simulink model "servomotor_pi_discreto"  (R2022b)
settings: Solver=FixedStepAuto  StartTime=0.0  StopTime=tempoSimulacao  FixedStep=1e-4  RelTol=1e-3
values from neighbouring files (symbols this model uses):
  controlador = projetarControladorPI(planta, requisitos)    [avaliarIndutor.m]    (also in avaliarTempoSubida.m)
  planta = obterPlantaServo()    [avaliarIndutor.m]    (also in avaliarTempoSubida.m)
undefined symbols (not defined in the file or in its folder): disturbio, referencia
settings Model: Creator=mmaximo  LastModifiedBy=danie
settings SolverCC: AlgebraicLoopSolver=TrustRegion
settings DebuggingCC: UnconnectedInputMsg=warning  UnconnectedOutputMsg=warning  UnconnectedLineMsg=warning  SFMachineParentedDataDiag=warning
settings ModelReferenceCC: EnableRefExpFcnMdlSchedulingChecks=on
settings RTWCC: DLArmComputeVersion=19.05

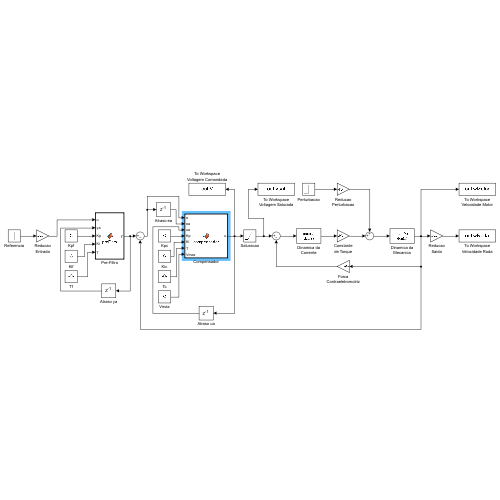
[thumbnail: Simulink's stored preview of the top-level diagram]
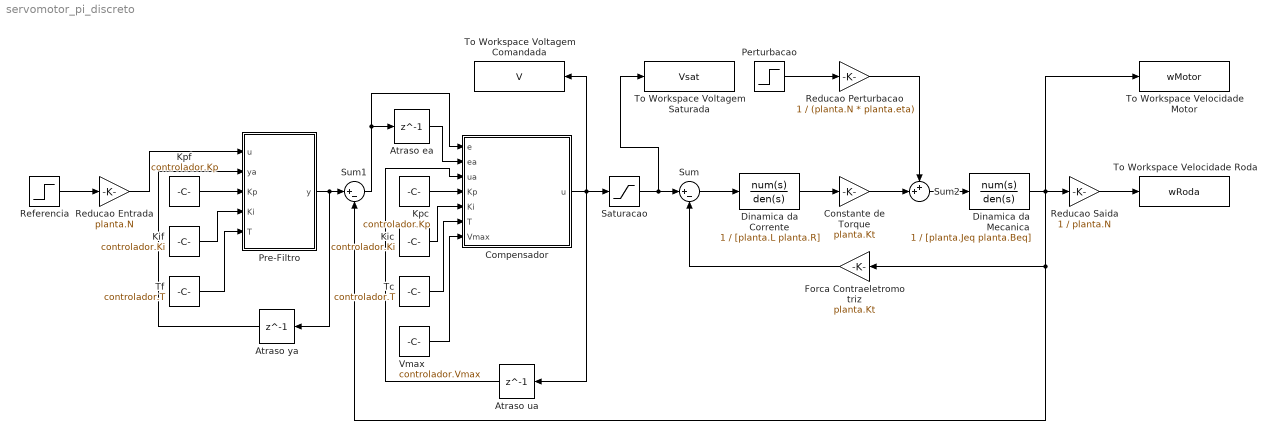
== system servomotor_pi_discreto ==
  Atraso ea : Delay  DelayLength=1  InitialCondition=0  SampleTime=controlador.T
  Atraso ua : Delay  DelayLength=1  InitialCondition=0  SampleTime=controlador.T
  Atraso ya : Delay  DelayLength=1  InitialCondition=0  SampleTime=controlador.T
  Compensador : MATLAB Function  TreatAsAtomicUnit=on  SystemSampleTime=controlador.T
  Constante de Torque : Gain  Gain=planta.Kt
  Dinamica da Corrente : TransferFcn  Numerator=1  Denominator=[planta.L planta.R]
  Dinamica da Mecanica : TransferFcn  Numerator=1  Denominator=[planta.Jeq planta.Beq]
  Forca Contraeletromotriz : Gain  Gain=planta.Kt
  Kic : Constant  Value=controlador.Ki
  Kif : Constant  Value=controlador.Ki
  Kpc : Constant  Value=controlador.Kp
  Kpf : Constant  Value=controlador.Kp
  Perturbacao : Step  Time=disturbio.instante  After=disturbio.amplitude  SampleTime=0
  Pre-Filtro : MATLAB Function  TreatAsAtomicUnit=on  SystemSampleTime=controlador.T
  Reducao Entrada : Gain  Gain=planta.N
  Reducao Perturbacao : Gain  Gain=1 / (planta.N * planta.eta)
  Reducao Saida : Gain  Gain=1 / planta.N
  Referencia : Step  Time=referencia.instante  After=referencia.amplitude  SampleTime=0
  Saturacao : Saturate  UpperLimit=planta.Vmax  LowerLimit=-planta.Vmax
  Sum : Sum  Inputs=|+-
  Sum1 : Sum  Inputs=|+-
  Sum2 : Sum  Inputs=++|
  Tc : Constant  Value=controlador.T
  Tf : Constant  Value=controlador.T
  To Workspace Velocidade Motor : ToWorkspace  VariableName=wMotor  SaveFormat=Structure With Time  SampleTime=1e-4
  To Workspace Velocidade Roda : ToWorkspace  VariableName=wRoda  SaveFormat=Structure With Time  SampleTime=1e-4
  To Workspace Voltagem Comandada : ToWorkspace  VariableName=V  SaveFormat=Structure With Time  SampleTime=1e-4
  To Workspace Voltagem Saturada : ToWorkspace  VariableName=Vsat  SaveFormat=Structure With Time  SampleTime=1e-4
  Vmax : Constant  Value=controlador.Vmax
  wires:
  Forca Contraeletromotriz/1 -> Sum/2
  Sum/1 -> Dinamica da Corrente/1
  Perturbacao/1 -> Reducao Perturbacao/1
  Dinamica da Corrente/1 -> Constante de Torque/1
  Dinamica da Mecanica/1 -> Reducao Saida/1, Sum1/2, Forca Contraeletromotriz/1, To Workspace Velocidade Motor/1
  Referencia/1 -> Reducao Entrada/1
  Reducao Saida/1 -> To Workspace Velocidade Roda/1
  Pre-Filtro/1(y) -> Atraso ya/1, Sum1/1
  Reducao Perturbacao/1 -> Sum2/1
  Constante de Torque/1 -> Sum2/2
  Sum2/1 -> Dinamica da Mecanica/1
  Compensador/1(u) -> Atraso ua/1, To Workspace Voltagem Comandada/1, Saturacao/1
  Sum1/1 -> Atraso ea/1, Compensador/1(e)
  Reducao Entrada/1 -> Pre-Filtro/1(u)
  Atraso ya/1 -> Pre-Filtro/2(ya)
  Kpf/1 -> Pre-Filtro/3(Kp)
  Kif/1 -> Pre-Filtro/4(Ki)
  Tf/1 -> Pre-Filtro/5(T)
  Atraso ea/1 -> Compensador/2(ea)
  Atraso ua/1 -> Compensador/3(ua)
  Kpc/1 -> Compensador/4(Kp)
  Kic/1 -> Compensador/5(Ki)
  Saturacao/1 -> To Workspace Voltagem Saturada/1, Sum/1
  Vmax/1 -> Compensador/7(Vmax)
  Tc/1 -> Compensador/6(T)

== matlab function servomotor_pi_discreto/Pre-Filtro ==
  data: u input; ya input; Kp input; Ki input; y output; T input
function y = preFiltro(u, ya, Kp, Ki, T)
% Implementa o pre-filtro discreto.
% Entradas:
% u: entrada atual u[k].
% ya: saida anterior y[k-1].
% Kp: ganho proporcional.
% Ki: ganho integrativo.
% T: tempo de amostragem.
% Saidas:
% y: saida atual y[k].

y = (ya + (Ki / Kp) * T * u) / (1 + (Ki / Kp) * T);

end

== matlab function servomotor_pi_discreto/Compensador ==
  data: e input; u output; ea input; ua input; Kp input; Ki input; T input; Vmax input
function u = compensador(e, ea, ua, Kp, Ki, T, Vmax)
% u = compensador(e, ea, ua, Kp, Ki, T, Vmax)
% Implementa o compensador PI discreto.
% Entradas:
% e: erro atual e[k].
% ea: erro anterior e[k-1].
% ua: comando anterior u[k-1].
% Kp: ganho proporcional.
% Ki: ganho integrativo.
% T: tempo de amostragem.
% Vmax: limite de tensao.
% Saidas:
% u: comando atual u[k].

u = ua + (Kp + Ki * T / 2) * e + (Ki * T / 2 - Kp) * ea;

% Anti-Windup
if u > Vmax
    u = Vmax;
elseif u < -Vmax
    u = -Vmax;
end

end
